simulink model "L0305"  (Simulink 9.1)
settings: Solver=ode45  StartTime=0.0  StopTime=30.0  MaxStep=0.01  RelTol=1e-3  EnableMultiTasking=on
libraries: simulink x2
settings Model: Creator=Irina  LastModifiedBy=Asus
settings DataIOCC: LimitDataPoints=on  SignalLoggingSaveFormat=ModelDataLogs
settings OptimizationCC: ExpressionDepthLimit=2147483647  InitFltsAndDblsToZero=on
settings DebuggingCC: SolverPrmCheckMsg=warning  FcnCallInpInsideContextMsg=warning  StateNameClashWarn=warning

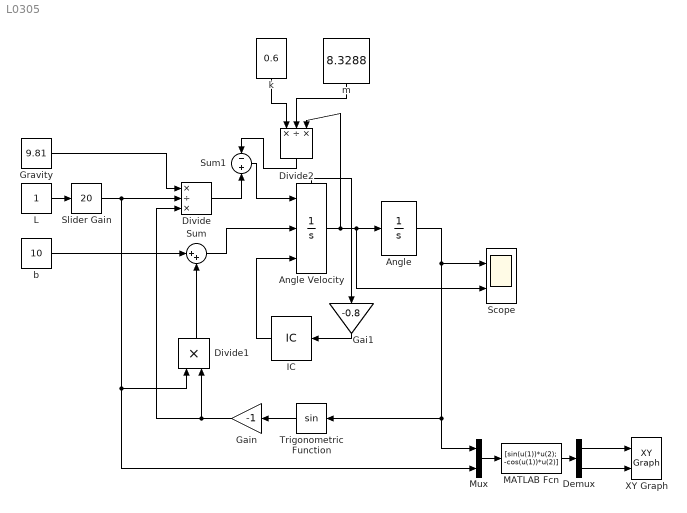
== system L0305 ==
  Angle : Integrator
  Angle Velocity : Integrator  ExternalReset=either  InitialConditionSource=external  InitialCondition=1  ShowStatePort=on
  Demux : Demux  Outputs=2
  Divide : Product  Inputs=*/*
  Divide1 : Product  Inputs=**
  Divide2 : Product  Inputs=*/*
  Gai1 : Gain  Gain=-0.8
  Gain : Gain  Gain=-1
  Gravity : Constant  Value=9.81
  IC : InitialCondition  Value=2
  L : Constant
  MATLAB Fcn : MATLABFcn  MATLABFcn=[sin(u(1))*u(2); -cos(u(1))*u(2)]
  Mux : Mux  Inputs=2
  Scope : Scope  NumInputPorts=2
  Slider Gain : simulink/Math Operations/Slider Gain  gain=20  low=0  high=50
  Sum : Sum  Inputs=|++
  Sum1 : Sum  Inputs=-+
  Trigonometric Function : Trigonometry
  XY Graph : simulink/Sinks/XY Graph  xmin=-35  xmax=35  ymin=-35  ymax=35  st=-1
  b : Constant  Value=10
  k : Constant  Value=0.6
  m : Constant  Value=8.3288
  wires:
  Angle Velocity/1 -> Angle/1, Scope/2, Divide2/3
  Gravity/1 -> Divide/1
  Trigonometric Function/1 -> Gain/1
  Angle/1 -> Scope/1, Trigonometric Function/1, Mux/1
  Gain/1 -> Divide/3, Divide1/2
  L/1 -> Slider Gain/1
  Mux/1 -> MATLAB Fcn/1
  MATLAB Fcn/1 -> Demux/1
  Demux/1 -> XY Graph/1
  Demux/2 -> XY Graph/2
  Slider Gain/1 -> Divide/2, Mux/2, Divide1/1
  Divide1/1 -> Sum/2
  b/1 -> Sum/1
  Sum/1 -> Angle Velocity/2
  IC/1 -> Angle Velocity/3
  Gai1/1 -> IC/1
  Angle Velocity/State -> Gai1/1
  m/1 -> Divide2/2
  k/1 -> Divide2/1
  Divide/1 -> Sum1/2
  Sum1/1 -> Angle Velocity/1
  Divide2/1 -> Sum1/1
